simulink model "REXduino_UNO_simulink"  (Simulink 7.8)
settings: Solver=FixedStepDiscrete  SolverMode=SingleTasking  StartTime=0.0  StopTime=600  FixedStep=0.1  RelTol=1e-3
libraries: logiclib x53, mathlib x34, anallib x8, genlib x4, reglib x2, speclib x1, execlib x1
settings Model: Creator=Jarda  LastModifiedBy=jsobota  ExtModeTrigMode=oneshot  ExtModeArmWhenConnect=off
settings DataIOCC: LimitDataPoints=off
settings OptimizationCC: BlockReduction=off  BooleanDataType=off
settings DebuggingCC: SaveWithParameterizedLinksMsg=none  SignalResolutionControl=TryResolveAllWithWarning  SolverPrmCheckMsg=none  MultiTaskDSMMsg=warning  MultiTaskCondExecSysMsg=none  StrictBusMsg=None
settings HardwareCC: TargetUnknown=on
settings RTWCC: IncludeERTFirstTime=on

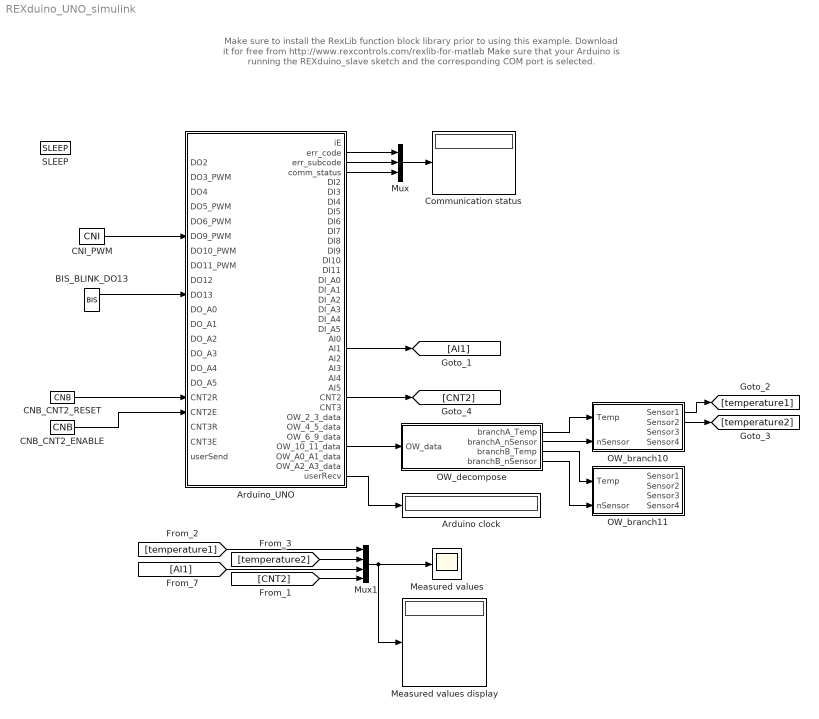
== system REXduino_UNO_simulink ==
  note: Make sure to install the RexLib function block library prior to using this example.
      | Download it for free from http://www.rexcontrols.com/rexlib-for-matlab
      |
      | Make sure that your Arduino is running the REXduino_slave sketch and the corresponding COM port is selected.
  Arduino clock : Display
  Arduino_UNO : Subsystem  mask(REX sequence){comPort=10, pinmode2=8: Counter, pinmode3=1: Not connected, pinmode4=10: Counter DIR / Encoder B, pinmode5=1: Not connected, pinmode6=1: Not connected, pinmode9=5: PWM (analog output), pinmode10=7: 1-Wire temperature, pinmode11=7: 1-Wire temperature, pinmodeA0=1: Not connected, pinmodeA1=6: Analog input, pinmodeA2=1: Not connected, pinmodeA3=1: Not connected, pinmodeA4=1: Not connected, pinmodeA5=1: Not connected}
      mask prompts: comPort "COM port number"; pinmode2 "Pin 2 mode"; pinmode3 "Pin 3 mode"; pinmode4 "Pin 4 mode"; pinmode5 "Pin 5 mode"; pinmode6 "Pin 6 mode"; pinmode9 "Pin 9 mode"; pinmode10 "Pin 10 mode"; pinmode11 "Pin 11 mode"; pinmodeA0 "Analog pin A0 mode"; pinmodeA1 "Analog pin A1 mode"; pinmodeA2 "Analog pin A2 mode"; pinmodeA3 "Analog pin A3 mode"; pinmodeA4 "Analog pin A4 mode"; pinmodeA5 "Analog pin A5 mode"
      mask StyleString: popup(1|2|3|4|5|6|7|8|9|10|11|12),popup(1: Not connected|2: Digital output|3: Digital input|4: Digital input with internal pull-up|5: --- N/A for this pin ---|6: --- N/A for this pin ---|7: 1-Wire temperature|8: Counter|9: Encoder A),popup(1: Not connected|2: Digital output|3: Digital input|4: Digital input with internal pull-up|5: PWM (analog output)|6: --- N/A for this pin ---|7: 1-Wire temperature|8: Counter|9: Encoder A),popup(1: Not connected|2: Digital output|3: Digital input|4: Digital input with internal pull-up|5: --- N/A for this pin ---|6: --- N/A for this pin ---|7: 1-Wire temperature|8: --- N/A for this pin ---|9: --- N/A for this pin ---|10: Counter DIR / Encoder B),popup(1: Not connected|2: Digital output|3: Digital input|4: Digital input with internal pull-up|5: --- N/A for this pin ---|6: --- N/A for this pin ---|7: 1-Wire temperature|8: --- N/A for this pin ---|9: --- N/A for this pin ---|10: Counter DIR / Encoder B),popup(1: Not connected|2: Digital output|3: Digital input|4: Digital input with internal pull-up|5: PWM (analog output)|6: --- N/A for this pin ---|7: 1-Wire temperature),popup(1: Not connected|2: Digital output|3: Digital input|4: Digital input with internal pull-up|5: PWM (analog output)|6: --- N/A for this pin ---|7: 1-Wire temperature),popup(1: Not connected|2: Digital output|3: Digital input|4: Digital input with internal pull-up|5: PWM (analog output)|6: --- N/A for this pin ---|7: 1-Wire temperature),popup(1: Not connected|2: Digital output|3: Digital input|4: Digital input with internal pull-up|5: PWM (analog output)|6: --- N/A for this pin ---|7: 1-Wire temperature),popup(1: Not connected|2: Digital output|3: Digital input|4: Digital input with internal pull-up|5: --- N/A for this pin ---|6: Analog input|7: 1-Wire temperature),popup(1: Not connected|2: Digital output|3: Digital input|4: Digital input with internal pull-up|5: --- N/A for this pin ---|6: Analog input|7: 1-Wire temperature),popup(1: Not connected|2: Digital output|3: Digital input|4: Digital input with internal pull-up|5: --- N/A for this pin ---|6: Analog input|7: 1-Wire temperature),popup(1: Not connected|2: Digital output|3: Digital input|4: Digital input with internal pull-up|5: --- N/A for this pin ---|6: Analog input|7: 1-Wire temperature),popup(1: Not connected|2: Digital output|3: Digital input|4: Digital input with internal pull-up|5: --- N/A for this pin ---|6: Analog input|7: 1-Wire temperature),popup(1: Not connected|2: Digital output|3: Digital input|4: Digital input with internal pull-up|5: --- N/A for this pin ---|6: Analog input|7: 1-Wire temperature)
  BIS_BLINK_DO13 : genlib/BIS  Y0=off  t1=0.9  t2=1.0  t3=0  t4=4  t5=5  t6=6  t7=7  t8=8  RPT=on  bEdit=off
  CNB_CNT2_ENABLE : mathlib/CNB  YCN=on
  CNB_CNT2_RESET : mathlib/CNB  YCN=off
  CNI_PWM : mathlib/CNI  icn=128
  Communication status : Display
  Measured values : Scope
      settings: TimeRange=30  YMin=0  YMax=300
  Measured values display : Display
  Mux : Mux  Inputs=3
  Mux1 : Mux
  OW_branch10 : Subsystem
      mask Type: REX sequence
  OW_branch11 : Subsystem
      mask Type: REX sequence
  OW_decompose : Subsystem
      mask Type: REX sequence
  SLEEP : execlib/SLEEP  ts=0.1
  wires:
  Arduino_UNO/22(AI1) -> [AI1]
  Arduino_UNO/27(CNT2) -> [CNT2]
  Arduino_UNO/32(OW_10_11_data) -> OW_decompose/1(OW_data)
  BIS_BLINK_DO13/1 -> Arduino_UNO/10(DO13)
  CNB_CNT2_ENABLE/1 -> Arduino_UNO/18(CNT2E)
  CNB_CNT2_RESET/1 -> Arduino_UNO/17(CNT2R)
  CNI_PWM/1 -> Arduino_UNO/6(DO9_PWM)
  [CNT2] -> Mux1/4
  [temperature1] -> Mux1/1
  [temperature2] -> Mux1/2
  [AI1] -> Mux1/3
  OW_decompose/1(branchA_Temp) -> OW_branch10/1(Temp)
  OW_decompose/2(branchA_nSensor) -> OW_branch10/2(nSensor)
  OW_branch10/1(Sensor1) -> [temperature1]
  OW_branch10/2(Sensor2) -> [temperature2]
  OW_decompose/3(branchB_Temp) -> OW_branch11/1(Temp)
  OW_decompose/4(branchB_nSensor) -> OW_branch11/2(nSensor)
  Arduino_UNO/2(err_code) -> Mux/1
  Arduino_UNO/3(err_subcode) -> Mux/2
  Arduino_UNO/4(comm_status) -> Mux/3
  Mux/1 -> Communication status/1
  Mux1/1 -> Measured values/1, Measured values display/1
  Arduino_UNO/35(userRecv) -> Arduino clock/1

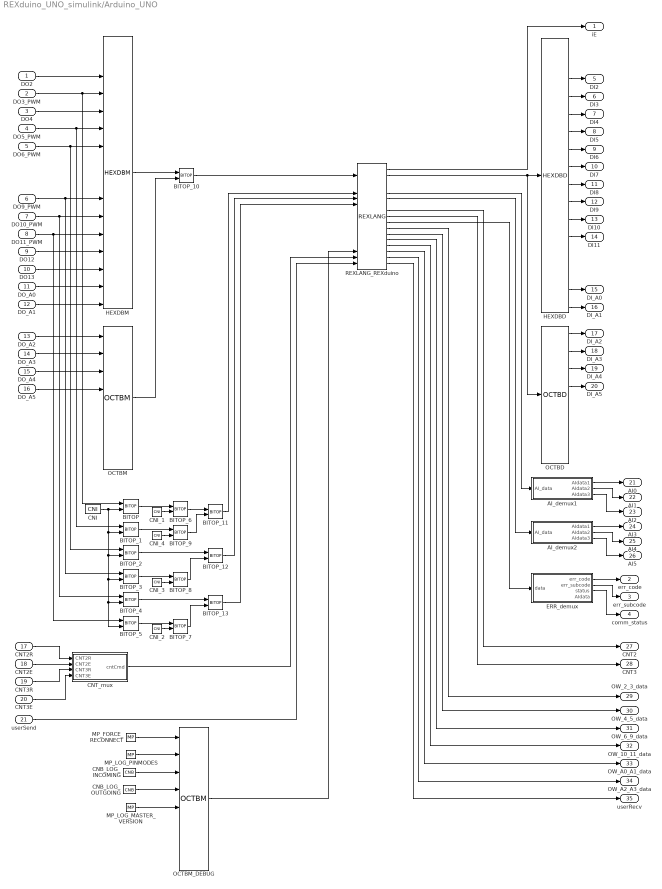
== system REXduino_UNO_simulink/Arduino_UNO ==
  DO2 : Inport
  DO3_PWM : Inport  Port=2
  DO4 : Inport  Port=3
  DO5_PWM : Inport  Port=4
  DO6_PWM : Inport  Port=5
  DO9_PWM : Inport  Port=6
  DO10_PWM : Inport  Port=7
  DO11_PWM : Inport  Port=8
  DO12 : Inport  Port=9
  DO13 : Inport  Port=10
  DO_A0 : Inport  Port=11
  DO_A1 : Inport  Port=12
  DO_A2 : Inport  Port=13
  DO_A3 : Inport  Port=14
  DO_A4 : Inport  Port=15
  DO_A5 : Inport  Port=16
  CNT2R : Inport  Port=17
  CNT2E : Inport  Port=18
  CNT3R : Inport  Port=19
  CNT3E : Inport  Port=20
  userSend : Inport  Port=21
  AI_demux1 : Subsystem
      mask Type: REX sequence
  AI_demux2 : Subsystem
      mask Type: REX sequence
  BITOP : logiclib/BITOP  iop=3: Bit AND
  BITOP_{1..5} (5 alike) : logiclib/BITOP  iop=3: Bit AND
  BITOP_{10..13} (4 alike) : logiclib/BITOP  iop=2: Bit OR
  BITOP_{6..9} (4 alike) : logiclib/BITOP  iop=5: Shift Left
  CNB_LOG_INCOMING : mathlib/CNB  YCN=off
  CNB_LOG_OUTGOING : mathlib/CNB  YCN=off
  CNI : mathlib/CNI  icn=255
  CNI_1 : mathlib/CNI  icn=8
  CNI_2 : mathlib/CNI  icn=8
  CNI_3 : mathlib/CNI  icn=24
  CNI_4 : mathlib/CNI  icn=24
  CNT_mux : Subsystem
      mask Type: REX sequence
  ERR_demux : Subsystem
      mask Type: REX sequence
  HEXDBD : logiclib/HEXDBD  shift=0
  HEXDBM : logiclib/HEXDBM  shift=0
  MP_FORCE_RECONNECT : genlib/MP  pwidth=10  BSTATE=off  RPTF=off
  MP_LOG_MASTER_VERSION : genlib/MP  pwidth=10  BSTATE=off  RPTF=off
  MP_LOG_PINMODES : genlib/MP  pwidth=10  BSTATE=off  RPTF=off
  OCTBD : logiclib/OCTBD  shift=16
  OCTBM : logiclib/OCTBM  shift=16
  OCTBM_DEBUG : logiclib/OCTBM  shift=0
  REXLANG_REXduino : speclib/REXLANG  tab_matlab=MORE  srcname=REXduino_master.stl  srctype=1: STL  stack=0  debug=1: No check  fname=REXduino_data.dat  p0=comPort  p1=pinmode2  p2=pinmode3  p3=pinmode4  p4=pinmode5  p5=pinmode6  p6=pinmode9  p7=pinmode10  p8=pinmode11  p9=pinmodeA0  p10=pinmodeA1  p11=pinmodeA2  p12=pinmodeA3  p13=pinmodeA4  p14=pinmodeA5  p15=1
  iE : Outport
  err_code : Outport  Port=2
  err_subcode : Outport  Port=3
  comm_status : Outport  Port=4
  DI2 : Outport  Port=5
  DI3 : Outport  Port=6
  DI4 : Outport  Port=7
  DI5 : Outport  Port=8
  DI6 : Outport  Port=9
  DI7 : Outport  Port=10
  DI8 : Outport  Port=11
  DI9 : Outport  Port=12
  DI10 : Outport  Port=13
  DI11 : Outport  Port=14
  DI_A0 : Outport  Port=15
  DI_A1 : Outport  Port=16
  DI_A2 : Outport  Port=17
  DI_A3 : Outport  Port=18
  DI_A4 : Outport  Port=19
  DI_A5 : Outport  Port=20
  AI0 : Outport  Port=21
  AI1 : Outport  Port=22
  AI2 : Outport  Port=23
  AI3 : Outport  Port=24
  AI4 : Outport  Port=25
  AI5 : Outport  Port=26
  CNT2 : Outport  Port=27
  CNT3 : Outport  Port=28
  OW_2_3_data : Outport  Port=29
  OW_4_5_data : Outport  Port=30
  OW_6_9_data : Outport  Port=31
  OW_10_11_data : Outport  Port=32
  OW_A0_A1_data : Outport  Port=33
  OW_A2_A3_data : Outport  Port=34
  userRecv : Outport  Port=35
  wires:
  AI_demux1/1(AIdata1) -> AI0/1
  AI_demux1/2(AIdata2) -> AI1/1
  AI_demux1/3(AIdata3) -> AI2/1
  AI_demux2/1(AIdata1) -> AI3/1
  AI_demux2/2(AIdata2) -> AI4/1
  AI_demux2/3(AIdata3) -> AI5/1
  BITOP/1 -> BITOP_6/1
  BITOP_1/1 -> BITOP_9/1
  BITOP_10/1 -> REXLANG_REXduino/2
  BITOP_11/1 -> REXLANG_REXduino/5
  BITOP_12/1 -> REXLANG_REXduino/6
  BITOP_13/1 -> REXLANG_REXduino/7
  BITOP_2/1 -> BITOP_12/1
  BITOP_3/1 -> BITOP_8/1
  BITOP_4/1 -> BITOP_13/1
  BITOP_5/1 -> BITOP_7/1
  BITOP_6/1 -> BITOP_11/1
  BITOP_7/1 -> BITOP_13/2
  BITOP_8/1 -> BITOP_12/2
  BITOP_9/1 -> BITOP_11/2
  CNI/1 -> BITOP/2, BITOP_1/2, BITOP_2/2, BITOP_3/2, BITOP_4/2, BITOP_5/2
  CNI_1/1 -> BITOP_6/2
  CNI_2/1 -> BITOP_7/2
  CNI_3/1 -> BITOP_8/2
  CNI_4/1 -> BITOP_9/2
  CNT2E/1 -> CNT_mux/2(CNT2E)
  CNT2R/1 -> CNT_mux/1(CNT2R)
  CNT3E/1 -> CNT_mux/4(CNT3E)
  CNT3R/1 -> CNT_mux/3(CNT3R)
  CNT_mux/1(cntCmd) -> REXLANG_REXduino/16
  DO10_PWM/1 -> BITOP_4/1, HEXDBM/11
  DO11_PWM/1 -> BITOP_5/1, HEXDBM/12
  DO12/1 -> HEXDBM/13
  DO13/1 -> HEXDBM/14
  DO2/1 -> HEXDBM/3
  DO3_PWM/1 -> BITOP/1, HEXDBM/4
  DO4/1 -> HEXDBM/5
  DO5_PWM/1 -> BITOP_1/1, HEXDBM/6
  DO6_PWM/1 -> BITOP_2/1, HEXDBM/7
  DO9_PWM/1 -> BITOP_3/1, HEXDBM/10
  DO_A0/1 -> HEXDBM/15
  DO_A1/1 -> HEXDBM/16
  DO_A2/1 -> OCTBM/1
  DO_A3/1 -> OCTBM/2
  DO_A4/1 -> OCTBM/3
  DO_A5/1 -> OCTBM/4
  ERR_demux/1(err_code) -> err_code/1
  ERR_demux/2(err_subcode) -> err_subcode/1
  ERR_demux/3(status) -> comm_status/1
  HEXDBD/3 -> DI2/1
  HEXDBD/4 -> DI3/1
  HEXDBD/5 -> DI4/1
  HEXDBD/6 -> DI5/1
  HEXDBD/7 -> DI6/1
  HEXDBD/8 -> DI7/1
  HEXDBD/9 -> DI8/1
  HEXDBD/10 -> DI9/1
  HEXDBD/11 -> DI10/1
  HEXDBD/12 -> DI11/1
  HEXDBD/15 -> DI_A0/1
  HEXDBD/16 -> DI_A1/1
  HEXDBM/1 -> BITOP_10/1
  OCTBD/1 -> DI_A2/1
  OCTBD/2 -> DI_A3/1
  OCTBD/3 -> DI_A4/1
  OCTBD/4 -> DI_A5/1
  OCTBM/1 -> BITOP_10/2
  REXLANG_REXduino/1 -> iE/1
  REXLANG_REXduino/2 -> HEXDBD/1, OCTBD/1
  REXLANG_REXduino/5 -> AI_demux1/1(AI_data)
  REXLANG_REXduino/6 -> AI_demux2/1(AI_data)
  REXLANG_REXduino/8 -> CNT2/1
  REXLANG_REXduino/9 -> CNT3/1
  REXLANG_REXduino/10 -> ERR_demux/1(data)
  REXLANG_REXduino/11 -> OW_2_3_data/1
  REXLANG_REXduino/12 -> OW_4_5_data/1
  REXLANG_REXduino/13 -> OW_6_9_data/1
  REXLANG_REXduino/14 -> OW_10_11_data/1
  REXLANG_REXduino/15 -> OW_A0_A1_data/1
  REXLANG_REXduino/16 -> OW_A2_A3_data/1
  REXLANG_REXduino/17 -> userRecv/1
  userSend/1 -> REXLANG_REXduino/17
  MP_FORCE_RECONNECT/1 -> OCTBM_DEBUG/1
  MP_LOG_PINMODES/1 -> OCTBM_DEBUG/2
  CNB_LOG_INCOMING/1 -> OCTBM_DEBUG/3
  CNB_LOG_OUTGOING/1 -> OCTBM_DEBUG/4
  OCTBM_DEBUG/1 -> REXLANG_REXduino/15
  MP_LOG_MASTER_VERSION/1 -> OCTBM_DEBUG/5

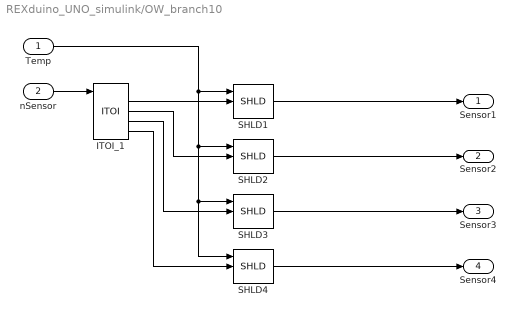
== system REXduino_UNO_simulink/OW_branch10 ==
  Temp : Inport
  nSensor : Inport  Port=2
  ITOI_1 : logiclib/ITOI  BINF=off  fktab=[0 1 2 4 8 0 0 0 0 0 0 0 0 0 0 0]
  SHLD{1..4} (4 alike) : anallib/SHLD  y0=0  mode=1: Triggered sampling
  Sensor1 : Outport
  Sensor2 : Outport  Port=2
  Sensor3 : Outport  Port=3
  Sensor4 : Outport  Port=4
  wires:
  ITOI_1/2 -> SHLD1/2
  ITOI_1/3 -> SHLD2/2
  ITOI_1/4 -> SHLD3/2
  ITOI_1/5 -> SHLD4/2
  SHLD1/1 -> Sensor1/1
  SHLD2/1 -> Sensor2/1
  SHLD3/1 -> Sensor3/1
  SHLD4/1 -> Sensor4/1
  Temp/1 -> SHLD3/1, SHLD4/1, SHLD2/1, SHLD1/1
  nSensor/1 -> ITOI_1/1

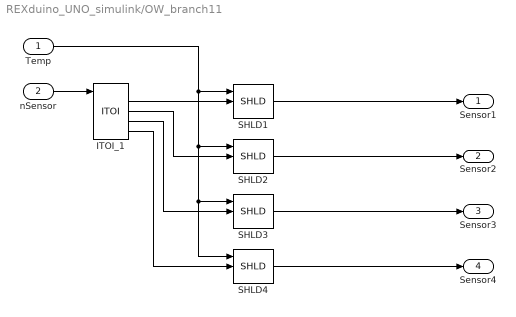
== system REXduino_UNO_simulink/OW_branch11 ==
  Temp : Inport
  nSensor : Inport  Port=2
  ITOI_1 : logiclib/ITOI  BINF=off  fktab=[0 1 2 4 8 0 0 0 0 0 0 0 0 0 0 0]
  SHLD{1..4} (4 alike) : anallib/SHLD  y0=0  mode=1: Triggered sampling
  Sensor1 : Outport
  Sensor2 : Outport  Port=2
  Sensor3 : Outport  Port=3
  Sensor4 : Outport  Port=4
  wires:
  ITOI_1/2 -> SHLD1/2
  ITOI_1/3 -> SHLD2/2
  ITOI_1/4 -> SHLD3/2
  ITOI_1/5 -> SHLD4/2
  SHLD1/1 -> Sensor1/1
  SHLD2/1 -> Sensor2/1
  SHLD3/1 -> Sensor3/1
  SHLD4/1 -> Sensor4/1
  Temp/1 -> SHLD3/1, SHLD4/1, SHLD2/1, SHLD1/1
  nSensor/1 -> ITOI_1/1

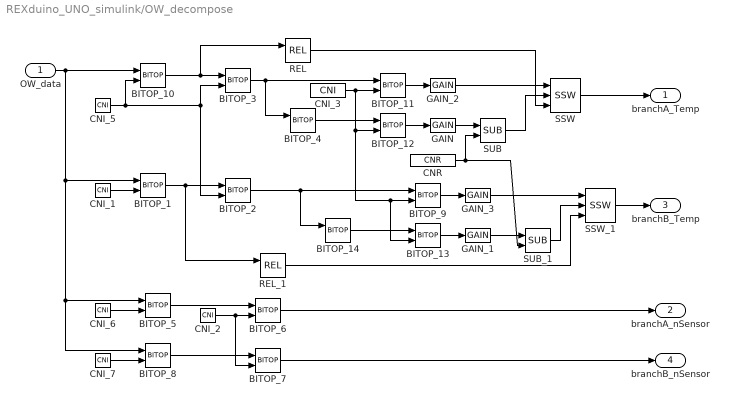
== system REXduino_UNO_simulink/OW_decompose ==
  OW_data : Inport
  BITOP_1 : logiclib/BITOP  iop=5: Shift Left
  BITOP_10 : logiclib/BITOP  iop=5: Shift Left
  BITOP_{6..7,9,11..13} (6 alike) : logiclib/BITOP  iop=3: Bit AND
  BITOP_14 : logiclib/BITOP  iop=1: Bit NOT
  BITOP_{2..3,5,8} (4 alike) : logiclib/BITOP  iop=6: Shift Right
  BITOP_4 : logiclib/BITOP  iop=1: Bit NOT
  CNI_1 : mathlib/CNI  icn=4
  CNI_2 : mathlib/CNI  icn=15
  CNI_3 : mathlib/CNI  icn=2047
  CNI_5 : mathlib/CNI  icn=20
  CNI_6 : mathlib/CNI  icn=12
  CNI_7 : mathlib/CNI  icn=28
  CNR : mathlib/CNR  ycn=0.0625
  GAIN : mathlib/GAIN  k=-0.0625
  GAIN_1 : mathlib/GAIN  k=-0.0625
  GAIN_2 : mathlib/GAIN  k=0.0625
  GAIN_3 : mathlib/GAIN  k=0.0625
  REL : mathlib/REL  irel=3: less than (<)
  REL_1 : mathlib/REL  irel=3: less than (<)
  SSW : reglib/SSW
  SSW_1 : reglib/SSW
  SUB : mathlib/SUB
  SUB_1 : mathlib/SUB
  branchA_Temp : Outport
  branchA_nSensor : Outport  Port=2
  branchB_Temp : Outport  Port=3
  branchB_nSensor : Outport  Port=4
  wires:
  BITOP_1/1 -> BITOP_2/1, REL_1/1
  BITOP_10/1 -> BITOP_3/1, REL/1
  BITOP_11/1 -> GAIN_2/1
  BITOP_12/1 -> GAIN/1
  BITOP_13/1 -> GAIN_1/1
  BITOP_14/1 -> BITOP_13/1
  BITOP_2/1 -> BITOP_14/1, BITOP_9/1
  BITOP_3/1 -> BITOP_11/1, BITOP_4/1
  BITOP_4/1 -> BITOP_12/1
  BITOP_5/1 -> BITOP_6/1
  BITOP_6/1 -> branchA_nSensor/1
  BITOP_7/1 -> branchB_nSensor/1
  BITOP_8/1 -> BITOP_7/1
  BITOP_9/1 -> GAIN_3/1
  CNI_1/1 -> BITOP_1/2
  CNI_2/1 -> BITOP_6/2, BITOP_7/2
  CNI_3/1 -> BITOP_11/2, BITOP_12/2, BITOP_13/2, BITOP_9/2
  CNI_5/1 -> BITOP_10/2, BITOP_2/2, BITOP_3/2
  CNI_6/1 -> BITOP_5/2
  CNI_7/1 -> BITOP_8/2
  CNR/1 -> SUB/2, SUB_1/2
  GAIN/1 -> SUB/1
  GAIN_1/1 -> SUB_1/1
  GAIN_2/1 -> SSW/1
  GAIN_3/1 -> SSW_1/1
  OW_data/1 -> BITOP_10/1, BITOP_1/1, BITOP_5/1, BITOP_8/1
  REL/1 -> SSW/3
  REL_1/1 -> SSW_1/3
  SSW/1 -> branchA_Temp/1
  SSW_1/1 -> branchB_Temp/1
  SUB/1 -> SSW/2
  SUB_1/1 -> SSW_1/2

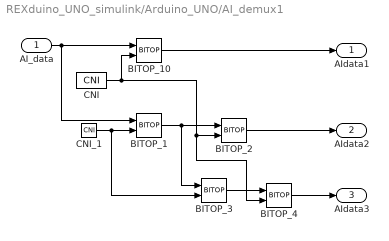
== system REXduino_UNO_simulink/Arduino_UNO/AI_demux1 ==
  AI_data : Inport
  BITOP_1 : logiclib/BITOP  iop=6: Shift Right
  BITOP_10 : logiclib/BITOP  iop=3: Bit AND
  BITOP_2 : logiclib/BITOP  iop=3: Bit AND
  BITOP_3 : logiclib/BITOP  iop=6: Shift Right
  BITOP_4 : logiclib/BITOP  iop=3: Bit AND
  CNI : mathlib/CNI  icn=1023
  CNI_1 : mathlib/CNI  icn=10
  AIdata1 : Outport
  AIdata2 : Outport  Port=2
  AIdata3 : Outport  Port=3
  wires:
  AI_data/1 -> BITOP_1/1, BITOP_10/1
  BITOP_1/1 -> BITOP_2/1, BITOP_3/1
  BITOP_10/1 -> AIdata1/1
  BITOP_2/1 -> AIdata2/1
  BITOP_3/1 -> BITOP_4/1
  BITOP_4/1 -> AIdata3/1
  CNI/1 -> BITOP_10/2, BITOP_2/2, BITOP_4/2
  CNI_1/1 -> BITOP_1/2, BITOP_3/2

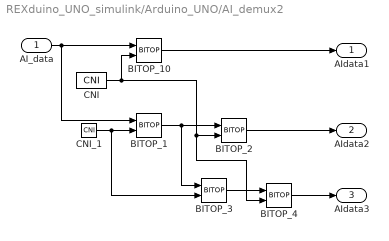
== system REXduino_UNO_simulink/Arduino_UNO/AI_demux2 ==
  AI_data : Inport
  BITOP_1 : logiclib/BITOP  iop=6: Shift Right
  BITOP_10 : logiclib/BITOP  iop=3: Bit AND
  BITOP_2 : logiclib/BITOP  iop=3: Bit AND
  BITOP_3 : logiclib/BITOP  iop=6: Shift Right
  BITOP_4 : logiclib/BITOP  iop=3: Bit AND
  CNI : mathlib/CNI  icn=1023
  CNI_1 : mathlib/CNI  icn=10
  AIdata1 : Outport
  AIdata2 : Outport  Port=2
  AIdata3 : Outport  Port=3
  wires:
  AI_data/1 -> BITOP_1/1, BITOP_10/1
  BITOP_1/1 -> BITOP_2/1, BITOP_3/1
  BITOP_10/1 -> AIdata1/1
  BITOP_2/1 -> AIdata2/1
  BITOP_3/1 -> BITOP_4/1
  BITOP_4/1 -> AIdata3/1
  CNI/1 -> BITOP_10/2, BITOP_2/2, BITOP_4/2
  CNI_1/1 -> BITOP_1/2, BITOP_3/2

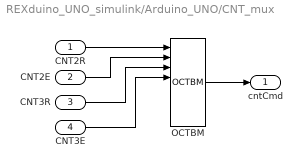
== system REXduino_UNO_simulink/Arduino_UNO/CNT_mux ==
  CNT2R : Inport
  CNT2E : Inport  Port=2
  CNT3R : Inport  Port=3
  CNT3E : Inport  Port=4
  OCTBM : logiclib/OCTBM  shift=0
  cntCmd : Outport
  wires:
  CNT2E/1 -> OCTBM/2
  CNT2R/1 -> OCTBM/1
  CNT3E/1 -> OCTBM/4
  CNT3R/1 -> OCTBM/3
  OCTBM/1 -> cntCmd/1

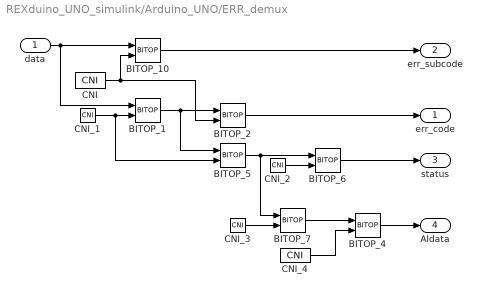
== system REXduino_UNO_simulink/Arduino_UNO/ERR_demux ==
  data : Inport
  BITOP_1 : logiclib/BITOP  iop=6: Shift Right
  BITOP_{2,4,6,10} (4 alike) : logiclib/BITOP  iop=3: Bit AND
  BITOP_5 : logiclib/BITOP  iop=6: Shift Right
  BITOP_7 : logiclib/BITOP  iop=6: Shift Right
  CNI : mathlib/CNI  icn=255
  CNI_1 : mathlib/CNI  icn=8
  CNI_2 : mathlib/CNI  icn=63
  CNI_3 : mathlib/CNI  icn=6
  CNI_4 : mathlib/CNI  icn=1023
  err_code : Outport
  err_subcode : Outport  Port=2
  status : Outport  Port=3
  AIdata : Outport  Port=4
  wires:
  BITOP_1/1 -> BITOP_2/1, BITOP_5/1
  BITOP_10/1 -> err_subcode/1
  BITOP_2/1 -> err_code/1
  BITOP_4/1 -> AIdata/1
  BITOP_5/1 -> BITOP_6/1, BITOP_7/1
  BITOP_6/1 -> status/1
  BITOP_7/1 -> BITOP_4/1
  CNI/1 -> BITOP_10/2, BITOP_2/2
  CNI_1/1 -> BITOP_1/2, BITOP_5/2
  CNI_2/1 -> BITOP_6/2
  CNI_3/1 -> BITOP_7/2
  CNI_4/1 -> BITOP_4/2
  data/1 -> BITOP_1/1, BITOP_10/1
